simulink model "Cart_Pendulum_Linearised_a_n9464263"  (R2020a)
settings: Solver=VariableStepAuto  StartTime=0.0  StopTime=10.0  RelTol=1e-3
values from neighbouring files (symbols this model uses):
  A = [ ... (first row only)    [MainFile_Linearised_a_n9464263.m]
  B = [ ... (first row only)    [MainFile_Linearised_a_n9464263.m]
settings Model: Creator=cal  LastModifiedBy=cal
settings DataIOCC: ExternalInput=[m M_c l g]  SaveFormat=Array

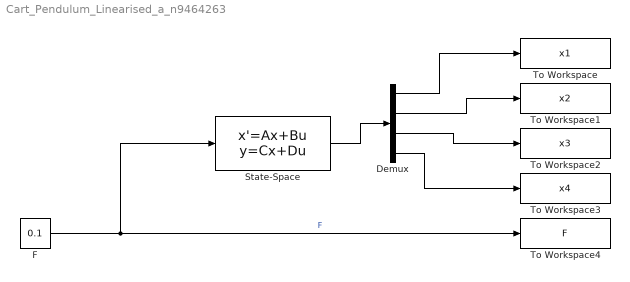
== system Cart_Pendulum_Linearised_a_n9464263 ==
  Demux : Demux
  F : Constant  Value=0.1
  State-Space : StateSpace  A=A  B=B  C=eye(4)  D=zeros([4 1])  InitialCondition=0
  To Workspace : ToWorkspace  VariableName=x1  SaveFormat=Timeseries  SampleTime=-1
  To Workspace1 : ToWorkspace  VariableName=x2  SaveFormat=Timeseries  SampleTime=-1
  To Workspace2 : ToWorkspace  VariableName=x3  SaveFormat=Timeseries  SampleTime=-1
  To Workspace3 : ToWorkspace  VariableName=x4  SaveFormat=Timeseries  SampleTime=-1
  To Workspace4 : ToWorkspace  VariableName=F  SaveFormat=Timeseries  SampleTime=-1
  wires:
  F/1 -> To Workspace4/1, State-Space/1  "F"
  State-Space/1 -> Demux/1
  Demux/1 -> To Workspace/1
  Demux/2 -> To Workspace1/1
  Demux/3 -> To Workspace2/1
  Demux/4 -> To Workspace3/1
